simulink model "PVModelPO"  (R2020a)
settings: Solver=VariableStepAuto  StartTime=0.0  StopTime=2  MaxStep=1e-4  RelTol=1e-3
libraries: powerlib x17, re_lib x5, powerlib_meascontrol x1
settings Model: Creator=Mahesh Krishna  LastModifiedBy=user
settings DataIOCC: ReturnWorkspaceOutputs=off
settings OptimizationCC: LifeSpan=inf
settings DebuggingCC: ArithmeticOperatorsInVariantConditions=warning
settings SFSimCC: SimUseLocalCustomCode=off  CustomCodeUndefinedFunction=UseInterfaceOnly
settings RTWCC: RTWUseLocalCustomCode=off
settings CodeAppCC: StateflowObjectComments=on
settings SimscapeCC: SimscapeNormalizeSystem=off

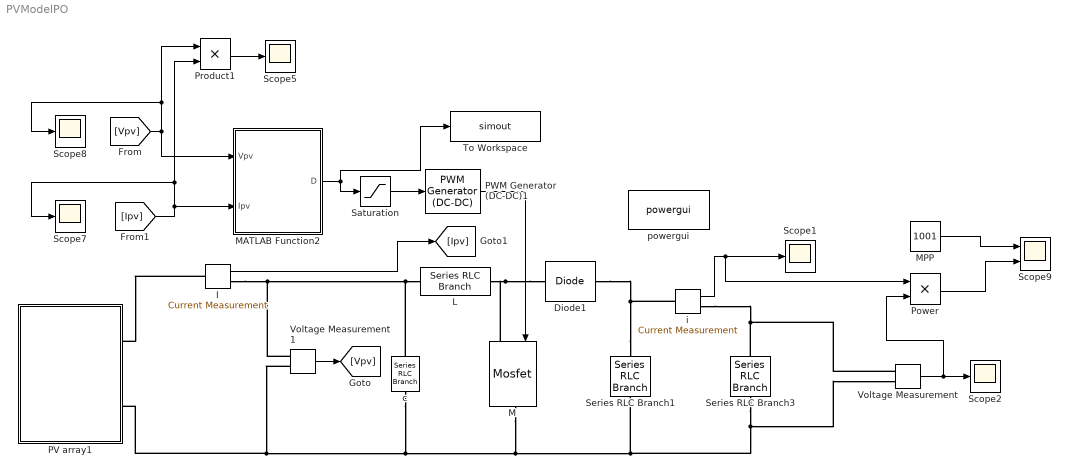
== system PVModelPO ==
  Diode1 : powerlib/Power Electronics/Diode  Ron=1e-3  Lon=0  Vf=0  IC=0  UseSnubber=off  Rs=inf  Cs=inf  Measurements=off
  I : powerlib/Measurements/Current Measurement  PhasorSimulation=off  OutputType=Magnitude  PSBequivalent=0
  L : powerlib/Elements/Series RLC Branch  LConnTagsString=__new0  RConnTagsString=__new0  BranchType=L  Resistance=1e-3  Inductance=5e-3  SetiL0=off  InitialCurrent=0  Capacitance=1e-6  Setx0=off  InitialVoltage=0  Measurements=None
  M : powerlib/Power Electronics/Mosfet  Ron=1e-3  Lon=0  Rd=1e-3  Vfd=0  IC=0  Rs=inf  Cs=inf  Measurements=off
  MATLAB Function2 : MATLAB Function  TreatAsAtomicUnit=on
  MPP : Constant  Value=1001
  PV array1 : Subsystem
  PWM Generator (DC-DC)1 : powerlib_meascontrol/Pulse & Signal Generators/PWM Generator (DC-DC)  Fsw=20000  Ts=0
  Power : Product
  Product1 : Product
  Saturation : Saturate  UpperLimit=1  LowerLimit=0
  Scope{1..2,5,7..8} (5 alike) : Scope
  Scope9 : Scope  NumInputPorts=2
  Series RLC Branch1 : powerlib/Elements/Series RLC Branch  LConnTagsString=__new0  RConnTagsString=__new0  BranchType=C  Resistance=1e-4  Inductance=200e-6  SetiL0=off  InitialCurrent=0  Capacitance=22e-6  Setx0=off  InitialVoltage=40  Measurements=None
  Series RLC Branch3 : powerlib/Elements/Series RLC Branch  LConnTagsString=__new0  RConnTagsString=__new0  BranchType=R  Resistance=100  Inductance=200e-6  SetiL0=off  InitialCurrent=0  Capacitance=1000e-6  Setx0=off  InitialVoltage=40  Measurements=None
  To Workspace : ToWorkspace  VariableName=simout  SampleTime=-1
  Voltage Measurement : powerlib/Measurements/Voltage Measurement  PhasorSimulation=off  OutputType=Magnitude  PSBequivalent=0
  Voltage Measurement1 : powerlib/Measurements/Voltage Measurement  PhasorSimulation=off  OutputType=Magnitude  PSBequivalent=0
  c : powerlib/Elements/Series RLC Branch  LConnTagsString=__new0  RConnTagsString=__new0  BranchType=C  Resistance=1e-3  Inductance=250e-6  SetiL0=off  InitialCurrent=0  Capacitance=2.2e-6  Setx0=off  InitialVoltage=0  Measurements=None
  i : powerlib/Measurements/Current Measurement  PhasorSimulation=off  OutputType=Magnitude  PSBequivalent=0
  powergui : powerlib/powergui  Priority=1  SimulationMode=Continuous  SampleTime=50e-6  frequency=60  Iterations=50  frequencyindice=0  Pbase=100e6  ErrMax=1e-4  UnitsV=kV  UnitsW=MW  buscounter=0  FunctionMessages=off  echomessages=off  EnableUseOfTLC=off  CurrentSourceSwitches=off  DisableSnubberDevices=off  DisableRonSwitches=off  DisableVfSwitches=off  DisplayEquations=off  AutomaticDiscreteSolvers=off  SolverType=Tustin/Backward Euler (TBE)  Interpol=off  ExternalGateDelay=off  methode=off  Ts=100  x0status=blocks  SPID=on  SwTol=0  HookPort=off  NonlinearTolerance=1e-4  nMaxIteration=100  ContinueOnMaxIteration=off  RestoreLinks=warning  ResistiveCurrentMeasurement=off  Frange=[0:2:500]  Ylog=off  Xlog=on  ShowGrid=off  save=off  variable=ZData  structure=0  ZoomFFT=off  StartTime=0.0  cycles=1  DisplayStyle=1  fundamental=60  FreqAxis=off  MaxFrequency=1000  frequencyindicesteady=1  RmsSteady=1  display=off
  wires:
  I/1 -> [Ipv]
  [Ipv] -> MATLAB Function2/2(Ipv), Scope7/1, Product1/2
  Voltage Measurement/1 -> Power/2, Scope2/1
  PWM Generator (DC-DC)1/1 -> M/1
  i/1 -> Power/1, Scope1/1
  Voltage Measurement1/1 -> [Vpv]
  [Vpv] -> MATLAB Function2/1(Vpv), Scope8/1, Product1/1
  Product1/1 -> Scope5/1
  MPP/1 -> Scope9/1
  Power/1 -> Scope9/2
  Saturation/1 -> PWM Generator (DC-DC)1/1
  MATLAB Function2/1(D) -> To Workspace/1, Saturation/1
  connections:
  i/RConn1 -- Series RLC Branch3/LConn1 -- Voltage Measurement/LConn1
  Series RLC Branch1/RConn1 -- Series RLC Branch3/RConn1 -- Voltage Measurement/LConn2 -- Voltage Measurement1/LConn2 -- PV array1/RConn2 -- c/RConn1 -- M/RConn1
  Series RLC Branch1/LConn1 -- Diode1/RConn1 -- i/LConn1
  I/LConn1 -- PV array1/RConn1
  Diode1/LConn1 -- M/LConn1 -- L/RConn1
  I/RConn1 -- Voltage Measurement1/LConn1 -- c/LConn1 -- L/LConn1

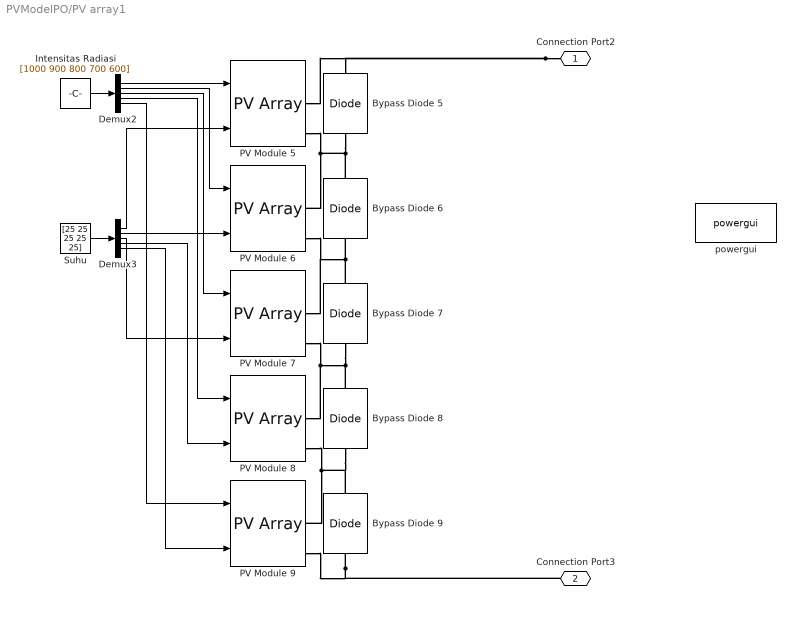
== system PVModelPO/PV array1 ==
  Bypass Diode {5..9} (5 alike) : powerlib/Power Electronics/Diode  Ron=0.001  Lon=0  Vf=0.8  IC=0  UseSnubber=off  Rs=500  Cs=250e-9  Measurements=off
  Demux2 : Demux  Outputs=5
  Demux3 : Demux  Outputs=5
  Intensitas Radiasi : Constant  Value=[1000 900 800 700 600]
  PV Module {5..9} (5 alike) : re_lib/Solar/PV Array  Npar=1  Nser=1  PlotType=array @ 1000 W/m2 & specified temperatures  S_vec="[ 1000  500  100 ]"  Temp_C_vec="[ 45 25  ]"  ModuleName=ET Solar Industry ET-P654200WW  PlotWhenSelected=off  Pm=200.2656  Ncell=54  Voc=32.72  Isc=7.86  Vm=27.21  Im=7.36  beta_Voc_pc=-0.35691  alpha_Isc_pc=0.050102  beta_Voc=-0.11678  alpha_Isc=0.003938  IL=7.8912  I0=2.3497e-10  nI=0.974  Rsh=176.8846  Rs=0.19523  RobustModel=off  RobustCellTemperature=25  BAL=off  Tc=1e-6  Tfilter=5e-5
  Suhu : Constant  Value=[25 25 25 25 25]
  powergui : powerlib/powergui  Priority=1  SimulationMode=Continuous  SampleTime=50e-6  frequency=60  Iterations=50  frequencyindice=0  Pbase=100e6  ErrMax=1e-4  UnitsV=kV  UnitsW=MW  buscounter=0  FunctionMessages=off  echomessages=off  EnableUseOfTLC=off  CurrentSourceSwitches=off  DisableSnubberDevices=off  DisableRonSwitches=off  DisableVfSwitches=off  DisplayEquations=off  AutomaticDiscreteSolvers=off  SolverType=Tustin/Backward Euler (TBE)  Interpol=off  ExternalGateDelay=off  methode=off  Ts=100  x0status=blocks  SPID=on  SwTol=0  HookPort=off  NonlinearTolerance=1e-4  nMaxIteration=100  ContinueOnMaxIteration=off  RestoreLinks=warning  ResistiveCurrentMeasurement=off  Frange=[0:2:500]  Ylog=off  Xlog=on  ShowGrid=off  save=off  variable=ZData  structure=0  ZoomFFT=off  StartTime=0.0  cycles=1  DisplayStyle=1  fundamental=60  FreqAxis=off  MaxFrequency=1000  frequencyindicesteady=1  RmsSteady=1  display=off
  Connection Port2 : PMIOPort  Side=Right
  Connection Port3 : PMIOPort  Port=2  Side=Right
  wires:
  Demux2/1 -> PV Module 5/1
  Demux3/4 -> PV Module 8/2
  Demux3/1 -> PV Module 5/2
  Demux3/3 -> PV Module 7/2
  Demux2/5 -> PV Module 9/1
  Demux2/4 -> PV Module 8/1
  Demux2/3 -> PV Module 7/1
  Demux3/5 -> PV Module 9/2
  Intensitas Radiasi/1 -> Demux2/1
  Demux2/2 -> PV Module 6/1
  Suhu/1 -> Demux3/1
  Demux3/2 -> PV Module 6/2
  connections:
  Bypass Diode 6/RConn1 -- Bypass Diode 5/LConn1 -- PV Module 5/RConn2 -- PV Module 6/RConn1
  Connection Port2/RConn1 -- PV Module 5/RConn1 -- Bypass Diode 5/RConn1
  Bypass Diode 9/LConn1 -- Connection Port3/RConn1 -- PV Module 9/RConn2
  Bypass Diode 7/RConn1 -- Bypass Diode 6/LConn1 -- PV Module 7/RConn1 -- PV Module 6/RConn2
  PV Module 8/RConn2 -- PV Module 9/RConn1 -- Bypass Diode 8/LConn1 -- Bypass Diode 9/RConn1
  PV Module 7/RConn2 -- PV Module 8/RConn1 -- Bypass Diode 7/LConn1 -- Bypass Diode 8/RConn1

== matlab function PVModelPO/MATLAB Function2 ==
  settings: updateMethod=DISCRETE  sampleTime=1e-4
  data: Vpv input; D output; Ipv input
function D = PO(Vpv,Ipv)

%% inisialisasi variabel persistent
persistent iterasi counter voltage power duty;

maxiterasi = 30;
 
if(isempty(iterasi))
    iterasi=1;
end

if(isempty(counter))
    counter=1;
end

if(isempty(voltage))
    voltage = zeros(maxiterasi);
end

if(isempty(power))
    power = zeros(maxiterasi);
end

if(isempty(duty))
    duty = zeros(maxiterasi);
end

deltaawal = 0.9;
deltad=0.01;
%% evaluasi duty cycle
%duty cycle dievaluasi hingga 200 kali hingga mendapat nilai yang stabil
if(counter>=1 && counter<=200)
    if(iterasi==1)
        duty(iterasi) = deltaawal;
        D = duty(iterasi);
        counter=counter+1;
    else
        D = duty(iterasi);
        counter=counter+1;
    end
    return;
else
    iterasi = iterasi+1;
    deltavoltage = Vpv - voltage(iterasi-1);
    deltap=(Vpv*Ipv) - power(iterasi-1);
    if (deltap>0)
        if (deltavoltage>0)
            D=duty(iterasi-1)+deltad;
        else
            D=duty(iterasi-1)-deltad;
        end
    else
        if (deltavoltage>0)
            D=duty(iterasi-1)-deltad;
        else
            D=duty(iterasi-1)+deltad;
        end
    end
    duty(iterasi) = D;
    voltage(iterasi) = Vpv;
    power(iterasi) = Vpv*Ipv;
    counter = 2;
end
end
